simulink model "ueb1_1d"  (R2013a)
settings: Solver=ode4  StartTime=0.0  StopTime=60.0  FixedStep=h  RelTol=1e-3
values from neighbouring files (symbols this model uses):
  A = [-alpha 1;-2*beta*x(1)*x(2)-1 beta*(1-(x(1))^2)]    [aufg32d.m]    (also in wok.m = [0,1;-om0^2,-2*dvek(i)*om0])
undefined symbols (not defined in the file or in its folder): B, C, D
settings Model: Creator=isyssim2  LastModifiedBy=isyssim2

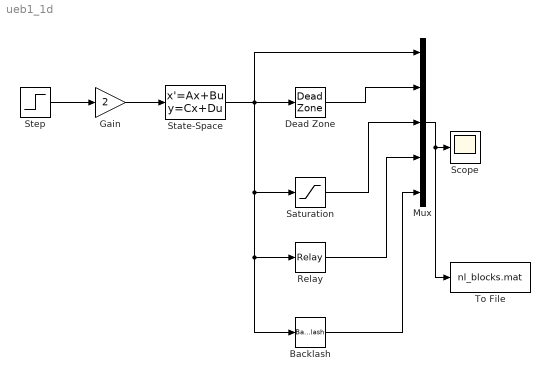
== system ueb1_1d ==
  Backlash : Backlash
  Dead Zone : DeadZone  SaturateOnIntegerOverflow=on
  Gain : Gain  Gain=2
  Mux : Mux  Inputs=5
  Relay : Relay
  Saturation : Saturate
  Scope : Scope
  State-Space : StateSpace  A=A  B=B  C=C  D=D
  Step : Step  SampleTime=0
  To File : ToFile  Filename=nl_blocks.mat
  wires:
  Step/1 -> Gain/1
  Gain/1 -> State-Space/1
  State-Space/1 -> Backlash/1, Relay/1, Saturation/1, Mux/1, Dead Zone/1
  Mux/1 -> Scope/1, To File/1
  Dead Zone/1 -> Mux/2
  Saturation/1 -> Mux/3
  Relay/1 -> Mux/4
  Backlash/1 -> Mux/5
